simulink model "pro2"  (R2020a)
settings: Solver=VariableStepAuto  StartTime=0.0  StopTime=10.0  RelTol=1e-3
model workspace (MAT data in the model file):
  b = Simulink.Parameter
  b.Value = 1000
  b.DataType = 'auto'
  b.Dimensions = [1 1]
  k1 = Simulink.Parameter
  k1.Value = 36000
  k1.DataType = 'auto'
  k1.Dimensions = [1 1]
  k2 = Simulink.Parameter
  k2.Value = 204034.4
  k2.DataType = 'auto'
  k2.Dimensions = [1 1]
  m1 = Simulink.Parameter
  m1.Value = 600
  m1.DataType = 'auto'
  m1.Dimensions = [1 1]
  m2 = Simulink.Parameter
  m2.Value = 90
  m2.DataType = 'auto'
  m2.Dimensions = [1 1]
settings Model: Creator=aa  LastModifiedBy=aa

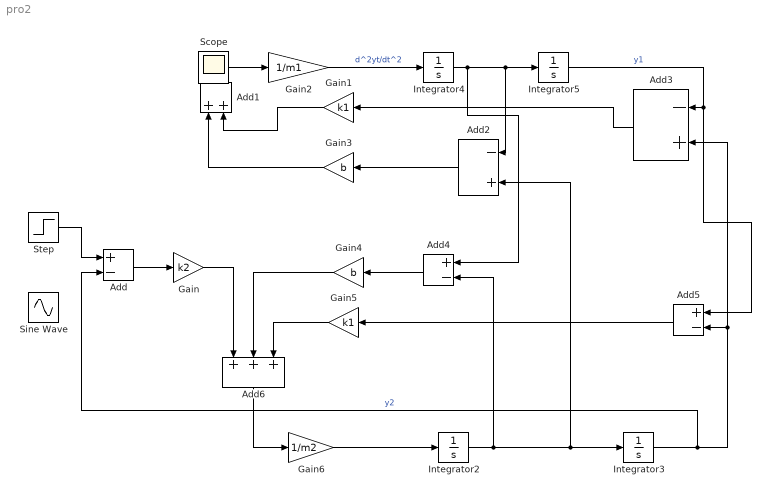
== system pro2 ==
  Add : Sum  Inputs=+-
  Add1 : Sum
  Add2 : Sum  Inputs=-+
  Add3 : Sum  Inputs=-+
  Add4 : Sum  Inputs=+-
  Add5 : Sum  Inputs=+-
  Add6 : Sum  Inputs=+++
  Gain : Gain  Gain=k2
  Gain1 : Gain  Gain=k1
  Gain2 : Gain  Gain=1/m1
  Gain3 : Gain  Gain=b
  Gain4 : Gain  Gain=b
  Gain5 : Gain  Gain=k1
  Gain6 : Gain  Gain=1/m2
  Integrator{2..5} (4 alike) : Integrator
  Sine Wave : Sin  SampleTime=0
  Step : Step  SampleTime=0
  Scope : Scope
  wires:
  Add4/1 -> Gain4/1
  Integrator2/1 -> Add4/2, Add2/2, Integrator3/1
  Add3/1 -> Gain1/1
  Add2/1 -> Gain3/1
  Add1/1 -> Gain2/1
  Integrator3/1 -> Add/2, Add5/2, Add3/2  "y2"
  Integrator5/1 -> Add5/1, Add3/1  "y1"
  Gain6/1 -> Integrator2/1
  Add6/1 -> Gain6/1
  Gain5/1 -> Add6/3
  Gain4/1 -> Add6/2
  Add5/1 -> Gain5/1
  Integrator4/1 -> Add4/1, Add2/1, Integrator5/1
  Gain3/1 -> Add1/1
  Gain2/1 -> Integrator4/1  "d^2yt/dt^2"
  Gain1/1 -> Add1/2
  Add/1 -> Gain/1
  Gain/1 -> Add6/1
  Step/1 -> Add/1
